simulink model "ANCbothpaths"  (R2023b)
settings: Solver=VariableStepAuto  StartTime=0.0  StopTime=20  RelTol=1e-3
libraries: dspadpt3 x3, audiosources x1
settings Model: Creator=aaron  LastModifiedBy=aaron

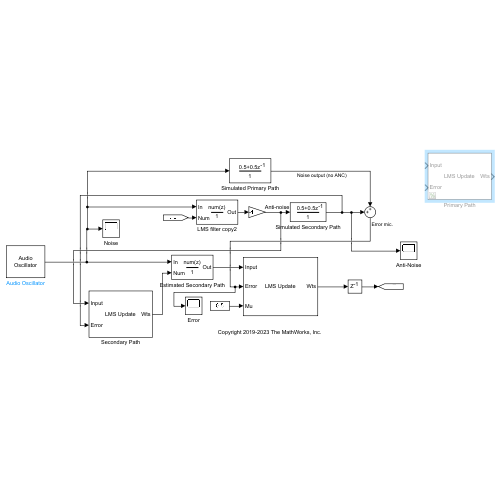
[thumbnail: Simulink's stored preview of the top-level diagram]
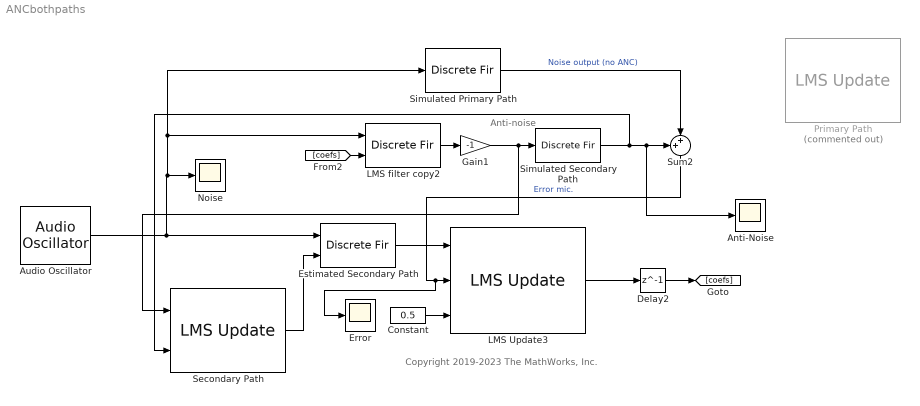
== system ANCbothpaths ==
  note: Anti-noise
  note: Copyright 2019-2023 The MathWorks, Inc.
  Anti-Noise : Scope
  Audio Oscillator : audiosources/Audio Oscillator  FrequencyPort=off  Frequency=300  AmplitudePort=off  Amplitude=30000  DCOffsetPort=off  PhaseOffset=0  DCOffset=0  WidthPort=off  Width=1  DutyCyclePort=off  DutyCycle=0.5  SampsPerFrame=1  Fs=44100  OutputDataType=double  SimulateUsing=Code generation
      settings: SignalType=sine
  Constant : Constant  Value=0.5
  Delay2 : Delay  DelayLength=1
  Error : Scope
  Estimated Secondary Path : DiscreteFir  CoefSource=Input port
      settings: InputPortMap=u0,u1
  Gain1 : Gain  Gain=-1
  LMS Update3 : dspadpt3/LMS Update  Method=Normalized LMS  Length=24  NumFilters=1  StepSizeSource=Input port  StepSize=0.1  LeakageFactor=1.0  InitialConditions=0  AdaptiveFilterMode=Tapped delay-line FIR filter  EnableAdaptInput=off  EnableResetInput=off  SimulateUsing=Interpreted execution
  LMS filter copy2 : DiscreteFir  CoefSource=Input port
      settings: InputPortMap=u0,u1
  Noise : Scope
  Primary Path : dspadpt3/LMS Update  Commented=on  Method=LMS  Length=L  NumFilters=1  StepSizeSource=Property  StepSize=0.001  LeakageFactor=1.0  InitialConditions=0  AdaptiveFilterMode=Tapped delay-line FIR filter  EnableAdaptInput=off  EnableResetInput=off  SimulateUsing=Code generation
  Secondary Path : dspadpt3/LMS Update  Method=LMS  Length=L  NumFilters=1  StepSizeSource=Property  StepSize=0.001  LeakageFactor=1.0  InitialConditions=0  AdaptiveFilterMode=Tapped delay-line FIR filter  EnableAdaptInput=off  EnableResetInput=off  SimulateUsing=Code generation
  Simulated Primary Path : DiscreteFir
  Simulated Secondary Path : DiscreteFir
  Sum2 : Sum  Inputs=++|
  wires:
  Audio Oscillator/1 -> Estimated Secondary Path/1, Simulated Primary Path/1, LMS filter copy2/1, Noise/1
  Simulated Secondary Path/1 -> Secondary Path/2, Anti-Noise/1, Sum2/1
  LMS filter copy2/1 -> Gain1/1
  Constant/1 -> LMS Update3/3
  LMS Update3/1 -> Delay2/1
  Estimated Secondary Path/1 -> LMS Update3/1
  [coefs] -> LMS filter copy2/2
  Sum2/1 -> Error/1, LMS Update3/2  "Error mic."
  Gain1/1 -> Secondary Path/1, Simulated Secondary Path/1
  Simulated Primary Path/1 -> Sum2/2  "Noise output (no ANC)"
  Delay2/1 -> [coefs]
  Secondary Path/1 -> Estimated Secondary Path/2
